simulink model "Seatblet_warning_system"  (R2025a)
settings: Solver=VariableStepAuto  StartTime=0.0  StopTime=20  RelTol=1e-3
settings Model: Creator=nikul  LastModifiedBy=nikul

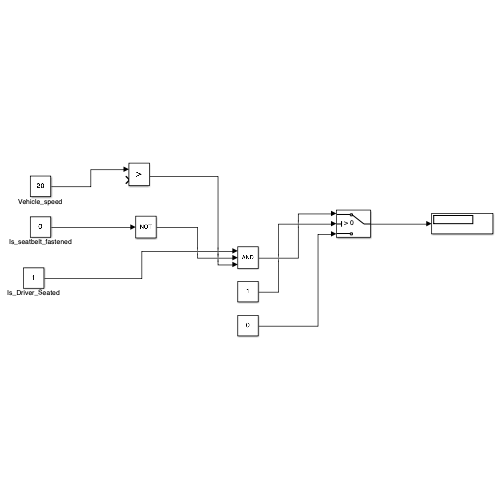
[thumbnail: Simulink's stored preview of the top-level diagram]
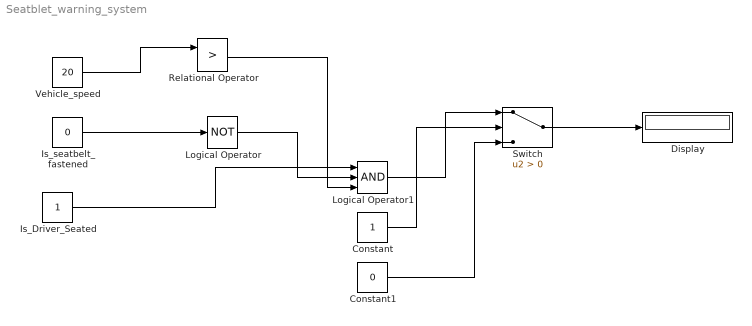
== system Seatblet_warning_system ==
  Constant : Constant
  Constant1 : Constant  Value=0
  Display : Display
  Is_Driver_Seated : Constant
  Is_seatbelt_fastened : Constant  Value=0
  Logical Operator : Logic  Operator=NOT  AllPortsSameDT=off  OutDataTypeStr=boolean
  Logical Operator1 : Logic  Inputs=3  AllPortsSameDT=off  OutDataTypeStr=boolean
  Relational Operator : RelationalOperator  Operator=>  OutDataTypeStr=boolean  RndMeth=Simplest  InputSameDT=off
  Switch : Switch  Criteria=u2 > Threshold  SaturateOnIntegerOverflow=off  InputSameDT=off
  Vehicle_speed : Constant  Value=20
  wires:
  Is_seatbelt_fastened/1 -> Logical Operator/1
  Vehicle_speed/1 -> Relational Operator/1
  Is_Driver_Seated/1 -> Logical Operator1/1
  Logical Operator/1 -> Logical Operator1/2
  Relational Operator/1 -> Logical Operator1/3
  Logical Operator1/1 -> Switch/1
  Constant/1 -> Switch/2
  Constant1/1 -> Switch/3
  Switch/1 -> Display/1
